simulink model "TSR_model"  (R2022b)
settings: Solver=VariableStepAuto  StartTime=0.0  StopTime=t_sample*n_sample  RelTol=1e-3
values from neighbouring files (symbols this model uses):
  air_den = 1.225    [wind_turbine_parameters.m]
  l1 = 56    [wind_turbine_parameters.m]
  lambda_op = 5.68    [wind_turbine_parameters.m]
  t_sample = 10*60    (= 600)    [wind_turbine_parameters.m]
libraries: spsWindTurbineLib x2, simulink x1
settings Model: Creator=luan  LastModifiedBy=marina

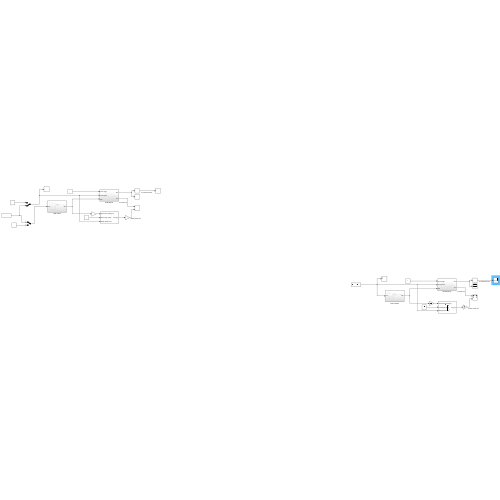
[thumbnail: Simulink's stored preview of the top-level diagram]
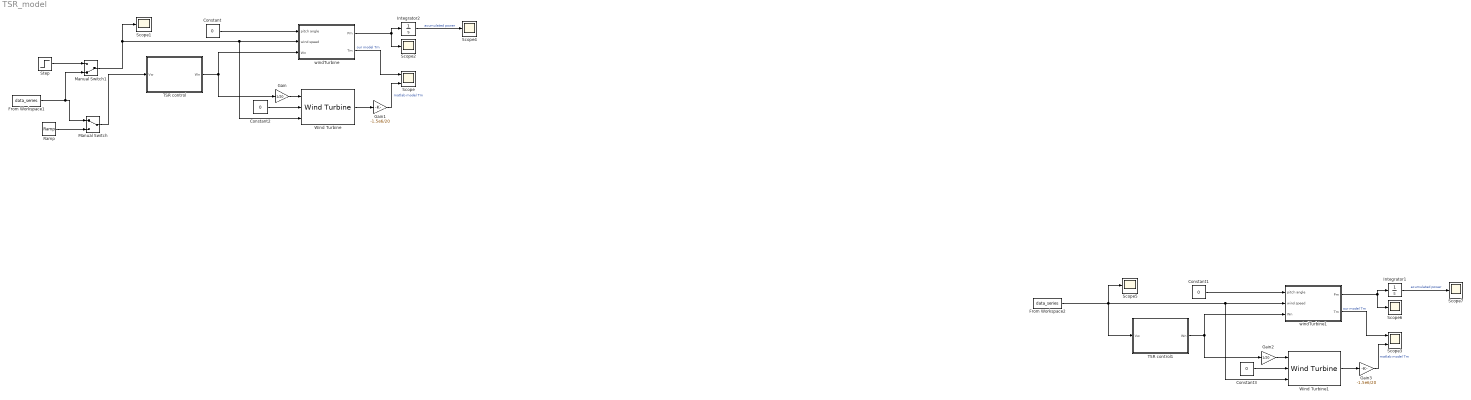
== system TSR_model ==
  Constant{,1..3} (4 alike) : Constant  Value=0
  From Workspace1 : FromWorkspace  VariableName=data_series  SampleTime=t_sample  OutputAfterFinalValue=Holding final value
  From Workspace2 : FromWorkspace  VariableName=data_series  SampleTime=t_sample  OutputAfterFinalValue=Holding final value
  Gain : Gain  Gain=1/20
  Gain1 : Gain  Gain=-1.5e6/20
  Gain2 : Gain  Gain=1/20
  Gain3 : Gain  Gain=-1.5e6/20
  Integrator1 : Integrator
  Integrator2 : Integrator
  Manual Switch : ManualSwitch
  Manual Switch1 : ManualSwitch  CurrentSetting=0
  Ramp : simulink/Sources/Ramp  slope=0.0001  start=0  InitialOutput=0.001
  Scope : Scope  NumInputPorts=2
  Scope{1..2,4..7} (6 alike) : Scope
  Scope3 : Scope  NumInputPorts=2
  Step : Step  Time=0  After=20  SampleTime=0
  TSR control : Subsystem
  TSR control1 : Subsystem
  Wind Turbine : spsWindTurbineLib/Wind Turbine  Pnom=1.5e6  Pelec_base=1.5e6/0.9  wind_base=4  P_wind_base=0.73  speed_nom=1.2  pitch_angle=0  c1_c6="[0.51763          116          0.4            5           21     0.006795]"  cp_nom=0.48  lambda_nom=8.1
  Wind Turbine1 : spsWindTurbineLib/Wind Turbine  Pnom=1.5e6  Pelec_base=1.5e6/0.9  wind_base=4  P_wind_base=0.73  speed_nom=1.2  pitch_angle=0  c1_c6="[0.51763          116          0.4            5           21     0.006795]"  cp_nom=0.48  lambda_nom=8.1
  windTurbine : Subsystem
  windTurbine1 : Subsystem
  wires:
  Step/1 -> Manual Switch1/1
  TSR control/1(Wn) -> windTurbine/3(Wn), Gain/1
  Ramp/1 -> Manual Switch/2
  Manual Switch1/1 -> Wind Turbine/3, windTurbine/2(wind speed), Scope1/1
  From Workspace1/1 -> Manual Switch/1, Manual Switch1/2
  Integrator2/1 -> Scope4/1  "acumulated power"
  Gain/1 -> Wind Turbine/1
  Gain1/1 -> Scope/2  "matlab model Tm"
  Constant2/1 -> Wind Turbine/2
  Manual Switch/1 -> TSR control/1(Vw)
  Constant/1 -> windTurbine/1(pitch angle)
  windTurbine/2(Tm) -> Scope/1  "our model Tm"
  Wind Turbine/1 -> Gain1/1
  windTurbine/1(Pm) -> Integrator2/1, Scope2/1
  TSR control1/1(Wn) -> windTurbine1/3(Wn), Gain2/1
  From Workspace2/1 -> TSR control1/1(Vw), Wind Turbine1/3, windTurbine1/2(wind speed), Scope5/1
  Integrator1/1 -> Scope7/1  "acumulated power"
  Gain2/1 -> Wind Turbine1/1
  Gain3/1 -> Scope3/2  "matlab model Tm"
  Constant3/1 -> Wind Turbine1/2
  Constant1/1 -> windTurbine1/1(pitch angle)
  windTurbine1/2(Tm) -> Scope3/1  "our model Tm"
  Wind Turbine1/1 -> Gain3/1
  windTurbine1/1(Pm) -> Integrator1/1, Scope6/1

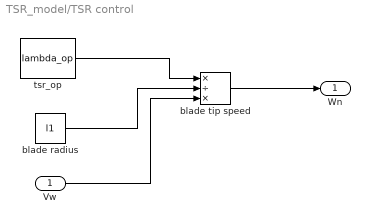
== system TSR_model/TSR control ==
  Vw : Inport
  blade radius : Constant  Value=l1
  blade tip speed : Product  Inputs=*/*
  tsr_op : Constant  Value=lambda_op
  Wn : Outport
  wires:
  blade tip speed/1 -> Wn/1
  Vw/1 -> blade tip speed/3
  tsr_op/1 -> blade tip speed/1
  blade radius/1 -> blade tip speed/2

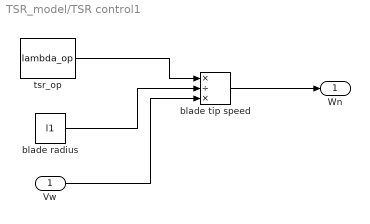
== system TSR_model/TSR control1 ==
  Vw : Inport
  blade radius : Constant  Value=l1
  blade tip speed : Product  Inputs=*/*
  tsr_op : Constant  Value=lambda_op
  Wn : Outport
  wires:
  blade tip speed/1 -> Wn/1
  Vw/1 -> blade tip speed/3
  tsr_op/1 -> blade tip speed/1
  blade radius/1 -> blade tip speed/2

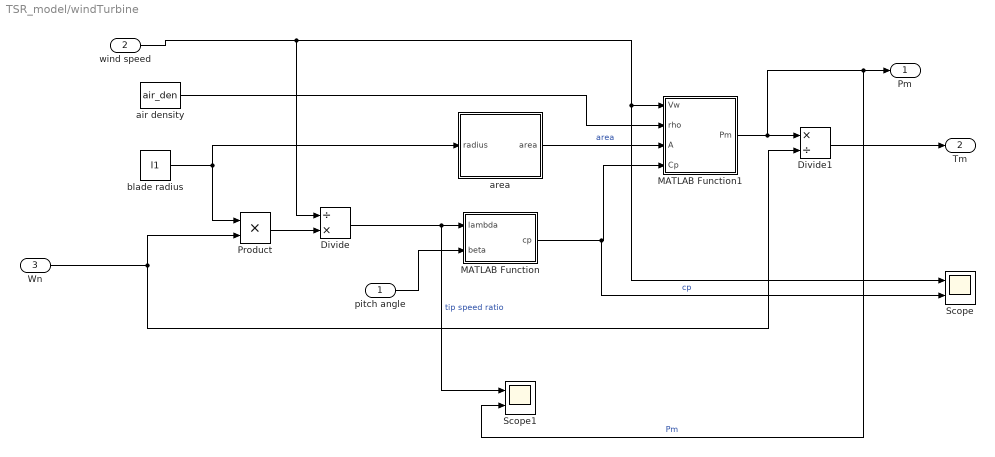
== system TSR_model/windTurbine ==
  pitch angle : Inport
  wind speed : Inport  Port=2
  Wn : Inport  Port=3
  Divide : Product  Inputs=/*
  Divide1 : Product  Inputs=*/
  MATLAB Function : MATLAB Function  TreatAsAtomicUnit=on
  MATLAB Function1 : MATLAB Function  TreatAsAtomicUnit=on
  Product : Product
  Scope : Scope  NumInputPorts=2
  Scope1 : Scope  NumInputPorts=2
  air density : Constant  Value=air_den
  area : Subsystem
  blade radius : Constant  Value=l1
  Pm : Outport
  Tm : Outport  Port=2
  wires:
  blade radius/1 -> Product/1, area/1(radius)
  Product/1 -> Divide/2
  wind speed/1 -> Scope/1, MATLAB Function1/1(Vw), Divide/1
  Divide/1 -> Scope1/1, MATLAB Function/1(lambda)  "tip speed ratio"
  pitch angle/1 -> MATLAB Function/2(beta)
  area/1(area) -> MATLAB Function1/3(A)  "area"
  MATLAB Function/1(cp) -> Scope/2, MATLAB Function1/4(Cp)  "cp"
  MATLAB Function1/1(Pm) -> Divide1/1, Scope1/2, Pm/1  "Pm"
  Divide1/1 -> Tm/1
  Wn/1 -> Divide1/2, Product/2
  air density/1 -> MATLAB Function1/2(rho)

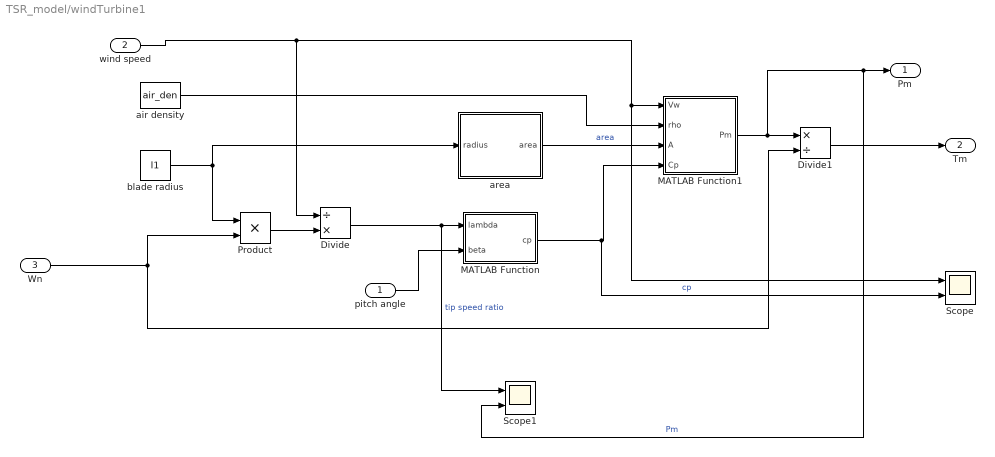
== system TSR_model/windTurbine1 ==
  pitch angle : Inport
  wind speed : Inport  Port=2
  Wn : Inport  Port=3
  Divide : Product  Inputs=/*
  Divide1 : Product  Inputs=*/
  MATLAB Function : MATLAB Function  TreatAsAtomicUnit=on
  MATLAB Function1 : MATLAB Function  TreatAsAtomicUnit=on
  Product : Product
  Scope : Scope  NumInputPorts=2
  Scope1 : Scope  NumInputPorts=2
  air density : Constant  Value=air_den
  area : Subsystem
  blade radius : Constant  Value=l1
  Pm : Outport
  Tm : Outport  Port=2
  wires:
  blade radius/1 -> Product/1, area/1(radius)
  Product/1 -> Divide/2
  wind speed/1 -> Scope/1, MATLAB Function1/1(Vw), Divide/1
  Divide/1 -> Scope1/1, MATLAB Function/1(lambda)  "tip speed ratio"
  pitch angle/1 -> MATLAB Function/2(beta)
  area/1(area) -> MATLAB Function1/3(A)  "area"
  MATLAB Function/1(cp) -> Scope/2, MATLAB Function1/4(Cp)  "cp"
  MATLAB Function1/1(Pm) -> Divide1/1, Scope1/2, Pm/1  "Pm"
  Divide1/1 -> Tm/1
  Wn/1 -> Divide1/2, Product/2
  air density/1 -> MATLAB Function1/2(rho)

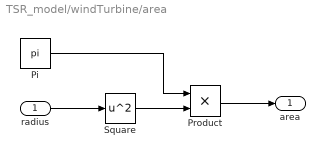
== system TSR_model/windTurbine/area ==
  radius : Inport
  Pi : Constant  Value=pi  OutDataTypeStr=Inherit: Inherit via back propagation
  Product : Product
  Square : Math  Operator=square
  area : Outport
  wires:
  radius/1 -> Square/1
  Square/1 -> Product/2
  Pi/1 -> Product/1
  Product/1 -> area/1

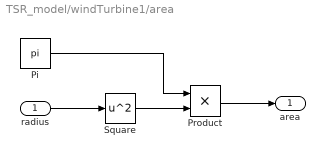
== system TSR_model/windTurbine1/area ==
  radius : Inport
  Pi : Constant  Value=pi  OutDataTypeStr=Inherit: Inherit via back propagation
  Product : Product
  Square : Math  Operator=square
  area : Outport
  wires:
  radius/1 -> Square/1
  Square/1 -> Product/2
  Pi/1 -> Product/1
  Product/1 -> area/1

== matlab function TSR_model/windTurbine/MATLAB Function1 ==
  data: Vw input; Pm output; rho input; A input; Cp input
function Pm = fcn(Vw, rho, A, Cp)

Pm = 0.5* Cp* rho* A* power(Vw, 3);

== matlab function TSR_model/windTurbine/MATLAB Function ==
  data: lambda input; cp output; beta input
function cp = fcn(lambda, beta)

k = load('coefficients.mat');
lambda_i =  1/(1/(lambda + 0.08*beta) - 0.035/(1+beta*beta*beta));

% Debug
% lambda_i
% k.k1 *(k.k2/lambda_i - k.k3*beta - k.k4*power(beta, k.k5) -k.k6)*exp(-k.k7/lambda_i)

cp = k.k1 *(k.k2/lambda_i - k.k3*beta - k.k4*power(beta, k.k5) -k.k6)*exp(-k.k7/lambda_i);

== matlab function TSR_model/windTurbine1/MATLAB Function ==
  data: lambda input; cp output; beta input
function cp = fcn(lambda, beta)

k = load('coefficients.mat');
lambda_i =  1/(1/(lambda + 0.08*beta) - 0.035/(1+beta*beta*beta));

% Debug
% lambda_i
% k.k1 *(k.k2/lambda_i - k.k3*beta - k.k4*power(beta, k.k5) -k.k6)*exp(-k.k7/lambda_i)

cp = k.k1 *(k.k2/lambda_i - k.k3*beta - k.k4*power(beta, k.k5) -k.k6)*exp(-k.k7/lambda_i);

== matlab function TSR_model/windTurbine1/MATLAB Function1 ==
  data: Vw input; Pm output; rho input; A input; Cp input
function Pm = fcn(Vw, rho, A, Cp)

Pm = 0.5* Cp* rho* A* power(Vw, 3);
